simulink library "DelayLibrary"  (R2022b)
settings: Solver=VariableStepAuto  StartTime=0.0  StopTime=10.0  RelTol=1e-3
undefined symbols (not defined in the file or in its folder): Column, delay_chain, L, max_delay, num_input_chs
libraries: FeaturePath x4, AudioStats x4, RTC x3, TuneVar x3, $bdroot x2, ITC x2, dspsigops x1, TOP x1
(part 2 of 2)

== matlab function DelayLibrary/PoolDelay/pool delay process ==
  data: u input; delayChain input; y output; variantSelect parameter; codeWorkMemory data_store_memory; delayBuffer data_store_memory; fastDelayBuffer data_store_memory
function y = pool_delay_process(u, delayChain, variantSelect)
% Pool delay function provides delay lines for N channels.  Core
% implementation provides delay of any positive integer value.  MDMA
% implementation provides integer value delays of a frame or greater. 
%
% Parameters:
%   u:              Input channels [frame size x number of inputs]
%   delayChain:     Delay in samples for each channel [1 x delay per channel]
%   variantSelect:  Variant selection of implementation (scaler)
%
% Global parameters:
%   delayBuffer:     Delay line circular buffer containing all channel  
%                    delay state data
%   fastDelayBuffer: Fast delay line circular buffer containing all channel  
%                    delay state data
%   codeWorkMemory:  Working memory set up during roommode reset/init CRL
%                    function call [1 x codeWorkMemorySize]

global delayBuffer;
global fastDelayBuffer;
global codeWorkMemory;

% Get the fast delay buffer sizes
delayBufferSize = numel(delayBuffer);
fastDelayBufferSize = numel(fastDelayBuffer);

% Set correct data types
delayChain = uint32(delayChain);
delayBufferSize = uint32(delayBufferSize);
fastDelayBufferSize = uint32(fastDelayBufferSize);

% There are three implementation types:
% Type       Value     Description
% L1 Memory    1       Optimized CRL C code using L1 memory delay buffer and 
%                      core for movement of data in/out of delay buffer
% L2 Memory    2       Optimized CRL C code using L2 memory delay buffer and
%                      MDMA for movement of data in/out of delay buffer
% Generic      3       Generic implementation for other targets without CRL

% Simulation
if(coder.target('MATLAB') || coder.target('Sfun')) 
    if (variantSelect == 2)
        % Simulation does not distribute delay state across two delay
        % buffers. It uses one delay buffer.
        y = PoolDelaySim(u, delayChain, ...
                         (fastDelayBufferSize + delayBufferSize));        
    else
        y = PoolDelaySim(u, delayChain, fastDelayBufferSize);
    end

% Code generation
else 
    if (variantSelect == 1)
        y = pool_delay_core_process(u, delayChain, codeWorkMemory);
    elseif (variantSelect == 2)
        y = pool_delay_mdma_process(u, delayChain, codeWorkMemory);
    else
        y = PoolDelayCodeGen(u, delayChain, fastDelayBufferSize);
    end  
end

end


% Pool delay CRL core step/process function conceptual specification
function y = pool_delay_core_process(u, delayChain, workMemory)
% If target == codegen, error out if no CRL found
coder.replace('-errorifnoreplacement');

[frameSize, numChannels] = size(u);
y = single(zeros(frameSize, numChannels));
end

% Pool delay CRL MDMA step/process function conceptual specification
function y = pool_delay_mdma_process(u, delayChain, workMemory)
% If target == codegen, error out if no CRL found
coder.replace('-errorifnoreplacement');

[frameSize, numChannels] = size(u);
y = single(zeros(frameSize, numChannels));
end
